simulink model "Designation_simulink"  (R2024b)
settings: Solver=FixedStepAuto  StartTime=0.0  StopTime=1  FixedStep=1/200  RelTol=1e-3
values from neighbouring files (symbols this model uses):
  dz = 28*(pi/180)    (= 0.488692190558)    [Designation_Loop_2ndTF.m]    (also in Designation_Loop_Design.m; Stabilization_Loop_Design.m)
  input_deg = 5    [Designation_Loop_2ndTF.m]    (also in Designation_Loop_Design.m; Stabilization_Loop_Design.m)
  Kd = (2*Zc*Wc - Pm) / Km    (= 1.79425597919)    [Designation_Loop_2ndTF.m]    (also in Designation_Loop_Design.m = 2.69488642049; Performance_graph.m = (2*Zc*Wc - Pm) / Km; desig_polePlacement.m = 2.26863468635; designation_validation.m = 1.7943)
  Km = 9.993    [Designation_Loop_2ndTF.m]    (also in Designation_Loop_Design.m; Performance_graph.m; Stabilization_Loop_Design.m = 13.55; desig_polePlacement.m = 13.55)
  Kp = Wc^2 / Km    (= 57.6403482438)    [Designation_Loop_2ndTF.m]    (also in Designation_Loop_Design.m = 72.951065746; Performance_graph.m = Wc^2 / Km; Stabilization_Loop_Design.m = 1.02878228782; desig_polePlacement.m = 75.5719557196)
  Pm = 10.87    [Designation_Loop_2ndTF.m]    (also in Designation_Loop_Design.m; Performance_graph.m; Stabilization_Loop_Design.m = 14.06; desig_polePlacement.m = 14.06)
  W_sat = 1400    [Designation_Loop_2ndTF.m]    (also in Designation_Loop_Design.m; Stabilization_Loop_Design.m)
settings Model: Creator=chaeeun  LastModifiedBy=chaeeun

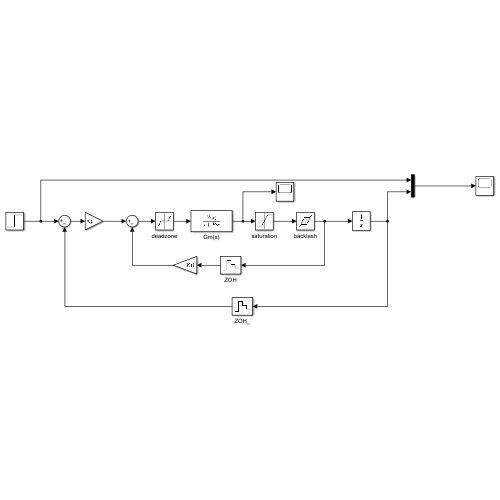
[thumbnail: Simulink's stored preview of the top-level diagram]
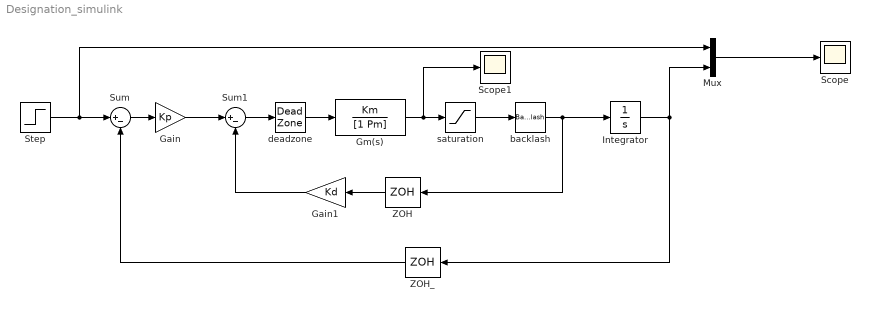
== system Designation_simulink ==
  Gain : Gain  Gain=Kp
  Gain1 : Gain  Gain=Kd
  Gm(s) : TransferFcn  Numerator=Km  Denominator=[1 Pm]
  Integrator : Integrator
  Mux : Mux  Inputs=2
  Scope : Scope
  Scope1 : Scope
  Step : Step  Time=0  After=input_deg  SampleTime=0  VectorParams1D=off
  Sum : Sum  Inputs=|+-
  Sum1 : Sum  Inputs=|+-
  ZOH : ZeroOrderHold  SampleTime=1/200
  ZOH_ : ZeroOrderHold  SampleTime=1/200
  backlash : Backlash  BacklashWidth=3
  deadzone : DeadZone  LowerValue=-dz  UpperValue=dz
  saturation : Saturate  UpperLimit=W_sat  LowerLimit=-W_sat
  wires:
  Sum/1 -> Gain/1
  Step/1 -> Mux/1, Sum/1
  Gain/1 -> Sum1/1
  Gain1/1 -> Sum1/2
  Mux/1 -> Scope/1
  Integrator/1 -> ZOH_/1, Mux/2
  ZOH/1 -> Gain1/1
  ZOH_/1 -> Sum/2
  Sum1/1 -> deadzone/1
  deadzone/1 -> Gm(s)/1
  backlash/1 -> ZOH/1, Integrator/1
  saturation/1 -> backlash/1
  Gm(s)/1 -> Scope1/1, saturation/1
